simulink model "ballInaHoop_getItUp"  (R2017a)
settings: Solver=ode45  StartTime=0.0  StopTime=3  MaxStep=1e-3  RelTol=1e-3  EnableMultiTasking=on
undefined symbols (not defined in the file): DiscIntNeverNeededParam, Kup, prms
libraries: simulink x5
settings Model: Creator=gurtnmar  LastModifiedBy=marti
settings SolverCC: AlgebraicLoopSolver=LineSearch
settings DataIOCC: LimitDataPoints=on  SaveFormat=Array
settings OptimizationCC: LifeSpan=inf
settings DebuggingCC: SFUnexpectedBacktrackingDiag=warning  SFNoUnconditionalDefaultTransitionDiag=warning  SFExecutionAtInitializationDiag=none
settings HardwareCC: ProdBitPerPointer=32  ProdBitPerSizeT=32  ProdBitPerPtrDiffT=32  ProdLargestAtomicFloat=None  ProdIntDivRoundTo=Undefined  ProdEndianess=Unspecified  ProdWordSize=32  ProdHWDeviceType=32-bit Generic
settings ModelReferenceCC: PropagateSignalLabelsOutOfModel=off
settings GRTTargetCC: TargetLangStandard=C89/C90 (ANSI)  GeneratePreprocessorConditionals=Disable all
settings ConfigComp: CovMetricSettings=dw  CovHtmlReporting=on  CovSaveCumulativeToWorkspaceVar=on  CovSaveSingleToWorkspaceVar=on  CovExternalEMLEnable=off

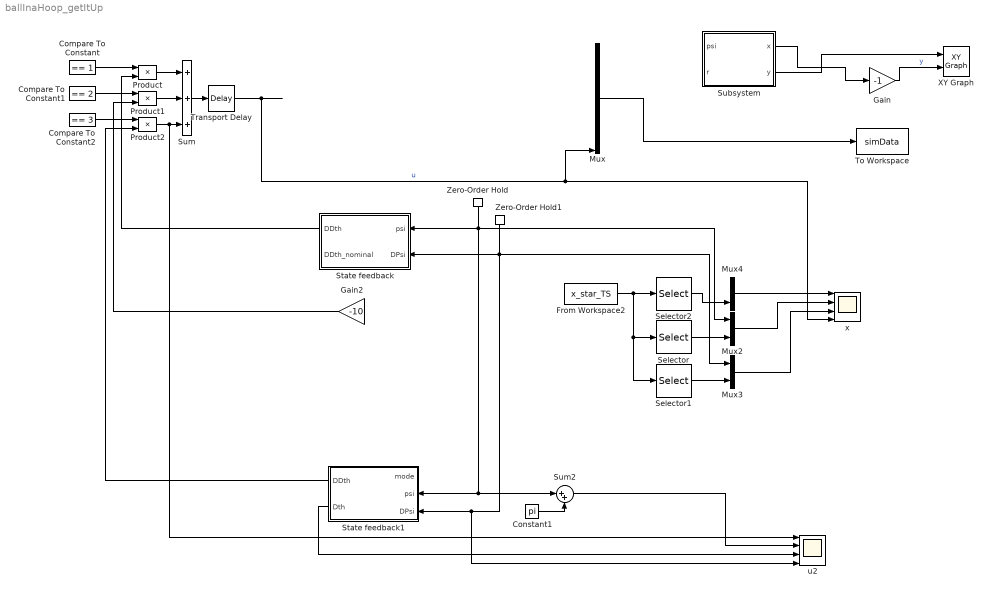
== system ballInaHoop_getItUp ==
  Compare To Constant : simulink/Logic and Bit Operations/Compare To Constant  relop===  const=1  OutDataTypeStr=boolean
  Compare To Constant1 : simulink/Logic and Bit Operations/Compare To Constant  relop===  const=2  OutDataTypeStr=boolean
  Compare To Constant2 : simulink/Logic and Bit Operations/Compare To Constant  relop===  const=3  OutDataTypeStr=boolean
  Constant1 : Constant  Value=pi
  From Workspace2 : FromWorkspace  VariableName=x_star_TS  SampleTime=prms.Ts  Interpolate=off  OutputAfterFinalValue=Setting to zero
  Gain : Gain  Gain=-1
  Gain2 : Gain  Gain=-10
  Mux : Mux  Inputs=9
  Mux2 : Mux  Inputs=2
  Mux3 : Mux  Inputs=2
  Mux4 : Mux  Inputs=2
  Product : Product
  Product1 : Product
  Product2 : Product
  Selector : Selector  InputPortWidth=3  IndexOptions=Index vector (dialog)  Indices=2  OutputSizes=1
  Selector1 : Selector  InputPortWidth=3  IndexOptions=Index vector (dialog)  Indices=3  OutputSizes=1
  Selector2 : Selector  InputPortWidth=3  IndexOptions=Index vector (dialog)  Indices=1  OutputSizes=1
  State feedback : Subsystem
  State feedback1 : Subsystem
  Subsystem : Subsystem
  Sum : Sum  Inputs=+++
  Sum2 : Sum  Inputs=|++
  To Workspace : ToWorkspace  VariableName=simData  SaveFormat=Timeseries  SampleTime=-1
  Transport Delay : TransportDelay  DelayTime=1/1000
  XY Graph : simulink/Sinks/XY Graph  xmin=-1.1*prms.Ro  xmax=1.1*prms.Ro  ymin=-1.1*prms.Ro  ymax=1.1*prms.Ro  st=-1
  Zero-Order Hold : ZeroOrderHold  SampleTime=prms.Ts
  Zero-Order Hold1 : ZeroOrderHold  SampleTime=prms.Ts
  u2 : Scope  NumInputPorts=4
  x : Scope  NumInputPorts=4
  wires:
  Gain/1 -> XY Graph/2  "y"
  Mux/1 -> To Workspace/1
  Subsystem/2(y) -> XY Graph/1
  Subsystem/1(x) -> Gain/1
  Transport Delay/1 -> Mux/9, x/4  "u"
  ? -> Mux/1  "th"
  ? -> Mux4/1, Gain2/1, Mux/2  "Dth"
  ? -> Zero-Order Hold/1, Subsystem/1(psi), Mux/3  "psi"
  ? -> Zero-Order Hold1/1, Mux/4  "Dpsi"
  ? -> Subsystem/2(r), Mux/5  "r"
  ? -> Mux/6  "Dr"
  ? -> Mux/7  "phi"
  ? -> Mux/8  "Dphi"
  State feedback/1(DDth) -> Product/2
  Sum/1 -> Transport Delay/1
  Zero-Order Hold1/1 -> Mux3/1, u2/4, State feedback1/3(DPsi), State feedback/2(DPsi)
  From Workspace2/1 -> Selector2/1, Selector1/1, Selector/1
  Selector/1 -> Mux2/2
  Selector1/1 -> Mux3/2
  Product/1 -> Sum/1
  Product1/1 -> Sum/2
  Product2/1 -> u2/1, Sum/3
  Compare To Constant/1 -> Product/1
  Compare To Constant1/1 -> Product1/1
  Compare To Constant2/1 -> Product2/1
  Zero-Order Hold/1 -> Mux2/1, State feedback1/2(psi), Sum2/1, State feedback/1(psi)
  State feedback1/1(DDth) -> Product2/2
  Constant1/1 -> Sum2/2
  Sum2/1 -> u2/2
  State feedback1/2(Dth) -> u2/3
  Mux4/1 -> x/1
  Mux2/1 -> x/2
  Mux3/1 -> x/3
  Selector2/1 -> Mux4/2
  Gain2/1 -> Product1/2
  ? -> State feedback1/1(mode), Compare To Constant2/1, Compare To Constant/1, Compare To Constant1/1

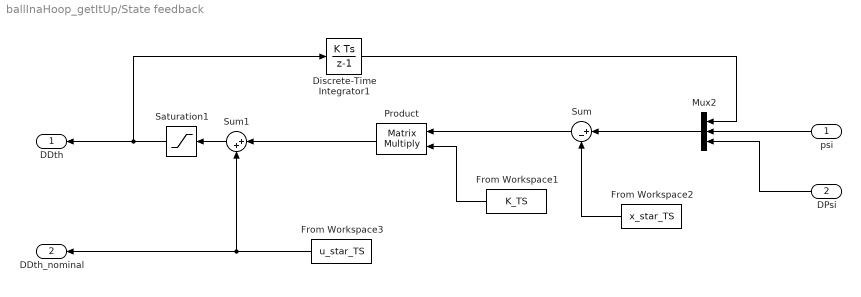
== system ballInaHoop_getItUp/State feedback ==
  psi : Inport
  DPsi : Inport  Port=2
  Discrete-Time Integrator1 : DiscreteIntegrator  InitialConditionSetting=State (most efficient)  SampleTime=prms.Ts  ICPrevOutput=DiscIntNeverNeededParam  ICPrevScaledInput=DiscIntNeverNeededParam
  From Workspace1 : FromWorkspace  VariableName=K_TS  SampleTime=prms.Ts  Interpolate=off  OutputAfterFinalValue=Setting to zero
  From Workspace2 : FromWorkspace  VariableName=x_star_TS  SampleTime=prms.Ts  Interpolate=off  OutputAfterFinalValue=Setting to zero
  From Workspace3 : FromWorkspace  VariableName=u_star_TS  SampleTime=prms.Ts  Interpolate=off  OutputAfterFinalValue=Setting to zero
  Mux2 : Mux  Inputs=3
  Product : Product  Multiplication=Matrix(*)
  Saturation1 : Saturate  UpperLimit=500  LowerLimit=-500
  Sum : Sum  Inputs=|+-
  Sum1 : Sum  Inputs=|++
  DDth : Outport
  DDth_nominal : Outport  Port=2
  wires:
  From Workspace1/1 -> Product/2
  Mux2/1 -> Sum/1
  From Workspace2/1 -> Sum/2
  Sum1/1 -> Saturation1/1
  Saturation1/1 -> Discrete-Time Integrator1/1, DDth/1
  Discrete-Time Integrator1/1 -> Mux2/1
  psi/1 -> Mux2/2
  DPsi/1 -> Mux2/3
  Product/1 -> Sum1/1
  From Workspace3/1 -> Sum1/2, DDth_nominal/1
  Sum/1 -> Product/1

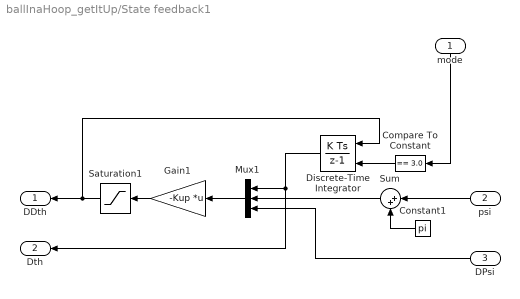
== system ballInaHoop_getItUp/State feedback1 ==
  mode : Inport
  psi : Inport  Port=2
  DPsi : Inport  Port=3
  Compare To Constant : simulink/Logic and Bit Operations/Compare To Constant  relop===  const=3.0  OutDataTypeStr=boolean
  Constant1 : Constant  Value=pi
  Discrete-Time Integrator : DiscreteIntegrator  ExternalReset=rising  InitialConditionSetting=State (most efficient)  SampleTime=1/50  ICPrevOutput=DiscIntNeverNeededParam  ICPrevScaledInput=DiscIntNeverNeededParam
  Gain1 : Gain  Gain=-Kup  Multiplication=Matrix(K*u)
  Mux1 : Mux  Inputs=3
  Saturation1 : Saturate  UpperLimit=prms.usat  LowerLimit=-prms.usat
  Sum : Sum  Inputs=|++
  DDth : Outport
  Dth : Outport  Port=2
  wires:
  Constant1/1 -> Sum/2
  Compare To Constant/1 -> Discrete-Time Integrator/2
  Sum/1 -> Mux1/2
  Mux1/1 -> Gain1/1
  mode/1 -> Compare To Constant/1
  psi/1 -> Sum/1
  Discrete-Time Integrator/1 -> Dth/1, Mux1/1
  DPsi/1 -> Mux1/3
  Gain1/1 -> Saturation1/1
  Saturation1/1 -> Discrete-Time Integrator/1, DDth/1

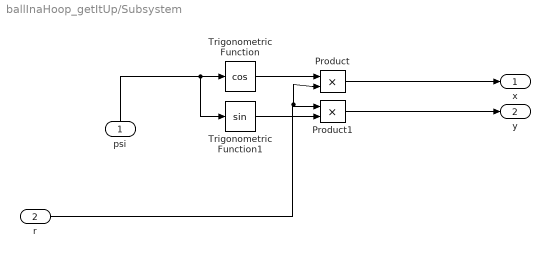
== system ballInaHoop_getItUp/Subsystem ==
  psi : Inport
  r : Inport  Port=2
  Product : Product
  Product1 : Product
  Trigonometric Function : Trigonometry  Operator=cos
  Trigonometric Function1 : Trigonometry
  x : Outport
  y : Outport  Port=2
  wires:
  Trigonometric Function/1 -> Product/1
  Product/1 -> x/1
  Product1/1 -> y/1
  Trigonometric Function1/1 -> Product1/2
  r/1 -> Product/2, Product1/1
  psi/1 -> Trigonometric Function1/1, Trigonometric Function/1
